simulink model "TARGET_CAN_WORKING_BUILD"  (R2023b)
settings: Solver=FixedStepAuto  StartTime=0.0  StopTime=Inf  RelTol=1e-3  EnableMultiTasking=on
InitFcn:
  | addpath('C:\MTU_DMD_CAN\COMMON_DATA'); mcb_pmsm_foc_qep_dyno_f28069m_data;
undefined symbols (not defined in the file): DiscIntNeverNeededParam, Down, GPTRIP1SEL, GPTRIP2SEL, inverter_motor1, inverter_motor2, PI_params_motor1, PI_params_motor2, pmsm_motor1, pmsm_motor2, PU_System_motor2, target, Ts, Ts_motor, Ts_speed, TZ1, TZ2, Up
libraries: simulink x11, c2802xlib x10, c280xlib x9, mcbcontrolslib x6, mcbpositiondecoderlib x6, c2806xlib x5, svdschedulerlib x3, mcbpmsmnonlinearlib x2, autolibpmsmexterior x2, mcbplantlib x2, demo_controls x1, slpidlib x1
(part 1 of 3)
settings Model: SimulationMode=external  ExtModeTrigDuration=8  Creator=The MathWorks, Inc.  LastModifiedBy=vmbasvi
settings OptimizationCC: DefaultParameterBehavior=Inlined  DefaultUnderspecifiedDataType=single  EnhancedBackFolding=on  PassReuseOutputArgsAs=Individual arguments  LifeSpan=Inf  MaxStackSize=1024  OptimizeBlockOrder=speed  DifferentSizesBufferReuse=on  OptimizationCustomize=off  EfficientTunableParamExpr=on
settings DebuggingCC: MultiTaskDSMMsg=none  ParameterPrecisionLossMsg=none  ParameterTunabilityLossMsg=error  ModelReferenceExtraNoncontSigs=none
settings HardwareCC: ProdBitPerChar=16  ProdBitPerInt=16  ProdBitPerPointer=32  ProdBitPerSizeT=32  ProdBitPerPtrDiffT=32  ProdLargestAtomicInteger=Integer  ProdLargestAtomicFloat=None  ProdWordSize=16  ProdLongLongMode=on  ProdHWDeviceType=Texas Instruments->C2000  HardwareBoardFeatureSet=SoCBlockset
settings ModelReferenceCC: ModelReferenceNumInstancesAllowed=Single
settings SFSimCC: MATLABDynamicMemAlloc=off
settings RTWCC: Description=Embedded Coder  SystemTargetFile=ert.tlc  HardwareBoard=TI Piccolo F28069M LaunchPad  TemplateMakefile=ert_default_tmf  Toolchain=Texas Instruments Code Composer Studio (C2000)  CodeProfilingSaveOptions=MetricsOnly
settings CodeAppCC: ForceParamTrailComments=on  IgnoreCustomStorageClasses=off  OperatorAnnotations=on  SimulinkDataObjDesc=on  SFDataObjDesc=on  InsertBlockDesc=on
settings ERTTargetCC: CodeReplacementLibrary=TI C28x  ParMdlRefBuildCompliant=off  CompOptLevelCompliant=off  ConcurrentExecutionCompliant=off  ExtModeTransport=4  ExtModeStaticAlloc=on  ExtModeAutomaticAllocSize=off  ExtModeStaticAllocSize=2000  ExtModeMexFile=ext_xcp  ExtModeIntrfLevel=Level2 - Open  MemSecPackage=tic2000demospkg

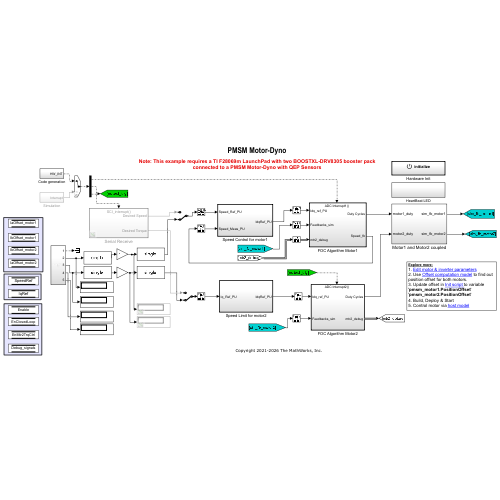
[thumbnail: Simulink's stored preview of the top-level diagram]
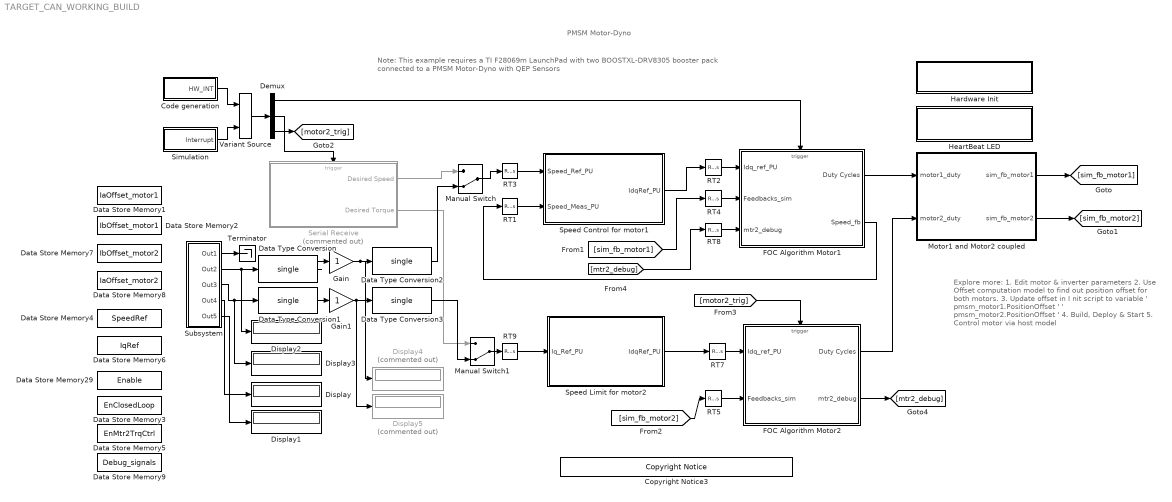
== system TARGET_CAN_WORKING_BUILD ==
  note: Explore more:
      | 1. Edit motor & inverter parameters
      | 2. Use Offset computation model to find out position offset for both motors.
      | 3. Update offset in I nit script to variable ' pmsm_motor1.PositionOffset '
      | ' pmsm_motor2.PositionOffset '
      | 4. Build, Deploy & Start
      | 5. Control motor via host model
  note: PMSM Motor-Dyno
  note: Note: This example requires a TI F28069m LaunchPad with two BOOSTXL-DRV8305 booster pack
      | connected to a PMSM Motor-Dyno with QEP Sensors
  Code generation : Subsystem
  Copyright Notice3 : demo_controls/Copyright Notice  year=2021  prod=tic2000
  Data Store Memory1 : DataStoreMemory  DataStoreName=IaOffset_motor1  ReadBeforeWriteMsg=warning  WriteAfterWriteMsg=warning  WriteAfterReadMsg=warning  InitialValue=inverter_motor1.CtSensAOffset  ShowAdditionalParam=off
  Data Store Memory2 : DataStoreMemory  DataStoreName=IbOffset_motor1  ReadBeforeWriteMsg=warning  WriteAfterWriteMsg=warning  WriteAfterReadMsg=warning  InitialValue=inverter_motor1.CtSensBOffset  ShowAdditionalParam=off
  Data Store Memory29 : DataStoreMemory  DataStoreName=Enable  ReadBeforeWriteMsg=warning  WriteAfterWriteMsg=warning  WriteAfterReadMsg=warning  ShowAdditionalParam=off  OutDataTypeStr=boolean
  Data Store Memory3 : DataStoreMemory  DataStoreName=EnClosedLoop  ReadBeforeWriteMsg=warning  WriteAfterWriteMsg=warning  WriteAfterReadMsg=warning  ShowAdditionalParam=off  OutDataTypeStr=boolean
  Data Store Memory4 : DataStoreMemory  DataStoreName=SpeedRef  ShowAdditionalParam=off
  Data Store Memory5 : DataStoreMemory  DataStoreName=EnMtr2TrqCtrl  ReadBeforeWriteMsg=warning  WriteAfterWriteMsg=warning  WriteAfterReadMsg=warning  ShowAdditionalParam=off  OutDataTypeStr=boolean
  Data Store Memory6 : DataStoreMemory  DataStoreName=IqRef  ShowAdditionalParam=off
  Data Store Memory7 : DataStoreMemory  DataStoreName=IbOffset_motor2  ReadBeforeWriteMsg=warning  WriteAfterWriteMsg=warning  WriteAfterReadMsg=warning  InitialValue=inverter_motor2.CtSensBOffset  ShowAdditionalParam=off
  Data Store Memory8 : DataStoreMemory  DataStoreName=IaOffset_motor2  ReadBeforeWriteMsg=warning  WriteAfterWriteMsg=warning  WriteAfterReadMsg=warning  InitialValue=inverter_motor2.CtSensBOffset  ShowAdditionalParam=off
  Data Store Memory9 : DataStoreMemory  DataStoreName=Debug_signals  ReadBeforeWriteMsg=warning  WriteAfterWriteMsg=warning  WriteAfterReadMsg=warning  InitialValue=5  ShowAdditionalParam=off  OutDataTypeStr=uint16
  Data Type Conversion{,1..3} (4 alike) : DataTypeConversion  OutDataTypeStr=single  SaturateOnIntegerOverflow=off  RndMeth=Floor
  Demux : Demux  Outputs=3
  Display{,1..3} (4 alike) : Display
  Display4 : Display  Commented=on
  Display5 : Display  Commented=on
  FOC Algorithm Motor1 : Subsystem
      settings: RTWSystemCode=Nonreusable function
  FOC Algorithm Motor2 : Subsystem
      settings: RTWSystemCode=Nonreusable function
  Gain : Gain
  Gain1 : Gain
  Hardware Init : Subsystem  TreatAsAtomicUnit=on
  HeartBeat LED : Subsystem
  Manual Switch : ManualSwitch  CurrentSetting=0
  Manual Switch1 : ManualSwitch  CurrentSetting=0
  Motor1 and Motor2 coupled : Subsystem
  RT1 : RateTransition  Deterministic=off  OutPortSampleTime=Ts_speed
  RT{2,4..5,7..8} (5 alike) : RateTransition  Deterministic=off
  RT3 : RateTransition  Deterministic=off  OutPortSampleTime=Ts_speed
  RT9 : RateTransition  Deterministic=off  OutPortSampleTime=Ts_speed
  Serial Receive : Subsystem  Commented=on  SystemSampleTime=1e-3
  Simulation : Subsystem
  Speed Control for motor1 : Subsystem  TreatAsAtomicUnit=on  SystemSampleTime=Ts_speed
  Speed Limit for motor2 : Subsystem  TreatAsAtomicUnit=on  SystemSampleTime=Ts_speed
  Subsystem : Subsystem
  Terminator : Terminator
  Variant Source : VariantSource  VariantControlMode=sim codegen switching  OutputFunctionCall=on
  wires:
  RT9/1 -> Speed Limit for motor2/1(Iq_Ref_PU)
  Motor1 and Motor2 coupled/2(sim_fb_motor2) -> [sim_fb_motor2]
  RT4/1 -> FOC Algorithm Motor1/2(Feedbacks_sim)
  RT7/1 -> FOC Algorithm Motor2/1(Idq_ref_PU)
  Speed Limit for motor2/1(IdqRef_PU) -> RT7/1
  Speed Control for motor1/1(IdqRef_PU) -> RT2/1
  Demux/3 -> [motor2_trig]
  [sim_fb_motor1] -> RT4/1
  RT1/1 -> Speed Control for motor1/2(Speed_Meas_PU)
  Demux/1 -> FOC Algorithm Motor1/Trigger
  [motor2_trig] -> FOC Algorithm Motor2/Trigger
  FOC Algorithm Motor2/1(Duty Cycles) -> Motor1 and Motor2 coupled/2(motor2_duty)
  Motor1 and Motor2 coupled/1(sim_fb_motor1) -> [sim_fb_motor1]
  [sim_fb_motor2] -> RT5/1
  RT5/1 -> FOC Algorithm Motor2/2(Feedbacks_sim)
  RT3/1 -> Speed Control for motor1/1(Speed_Ref_PU)
  Simulation/1(Interrupt) -> Variant Source/2
  FOC Algorithm Motor1/2(Speed_fb) -> RT1/1
  FOC Algorithm Motor1/1(Duty Cycles) -> Motor1 and Motor2 coupled/1(motor1_duty)
  Variant Source/1 -> Demux/1
  RT2/1 -> FOC Algorithm Motor1/1(Idq_ref_PU)
  Code generation/1(HW_INT) -> Variant Source/1
  Demux/2 -> Serial Receive/Trigger
  FOC Algorithm Motor2/2(mtr2_debug) -> [mtr2_debug]
  [mtr2_debug] -> RT8/1
  RT8/1 -> FOC Algorithm Motor1/3(mtr2_debug)
  Manual Switch1/1 -> RT9/1
  Subsystem/3(Out3) -> Display3/1, Data Type Conversion1/1
  Serial Receive/1(Desired Speed) -> Manual Switch/1
  Manual Switch/1 -> RT3/1
  Subsystem/2(Out2) -> Display2/1, Data Type Conversion/1
  Serial Receive/2(Desired Torque) -> Manual Switch1/1
  Subsystem/4(Out4) -> Display/1
  Subsystem/5(Out5) -> Display1/1
  Subsystem/1(Out1) -> Terminator/1
  Data Type Conversion/1 -> Gain/1
  Data Type Conversion1/1 -> Gain1/1
  Gain/1 -> Display4/1, Data Type Conversion2/1
  Data Type Conversion2/1 -> Manual Switch/2
  Gain1/1 -> Display5/1, Data Type Conversion3/1
  Data Type Conversion3/1 -> Manual Switch1/2

== system TARGET_CAN_WORKING_BUILD/Code generation ==
  HWI_ADCINT1 : svdschedulerlib/Hardware Interrupt v2  ISRGroup=ADC - Analog to Digital Converter  ISRName=ADCA1_INT  ISRNumber=32  NumEventsToServe=1  EventsList=[{'on','EOC event','1'};{'off','Overflow event','2'};{'off','Custom event','3'};{'off','Default event','4'}]  SelectedEvents={'event1'}  TaskPriority=30  DisablePreemption=off  ClearInterruptFlagsAtEndOfEvent=on  InterruptDefinitionFile=$(TARGET_ROOT)/registry/interrupts/F2837xS_interrupts.xml  HardwareBoard=F2837x  EnableSimPort=off
      settings: LibrarySourceBlock=c2000lib/Scheduling/Hardware Interrupt
  HWI_ADCINT2 : svdschedulerlib/Hardware Interrupt v2  ISRGroup=ADC - Analog to Digital Converter  ISRName=ADCA1_INT  ISRNumber=32  NumEventsToServe=1  EventsList={'on','EOC event','1';'off','Overflow event','2';'off','Custom event','3'}  SelectedEvents={'event1'}  TaskPriority=35  DisablePreemption=off  ClearInterruptFlagsAtEndOfEvent=on  InterruptDefinitionFile=$(TARGET_ROOT)/registry/interrupts/F2837xS_interrupts.xml  HardwareBoard=F2837x  EnableSimPort=off
      settings: LibrarySourceBlock=c2000lib/Scheduling/Hardware Interrupt
  HWI_SCIRXINTA : svdschedulerlib/Hardware Interrupt v2  Commented=on  ISRGroup=ADC - Analog to Digital Converter  ISRName=ADCA1_INT  ISRNumber=32  NumEventsToServe=1  EventsList={'on','EOC event','1';'off','Overflow event','2';'off','Custom event','3'}  SelectedEvents={'event1'}  TaskPriority=50  DisablePreemption=on  ClearInterruptFlagsAtEndOfEvent=on  InterruptDefinitionFile=$(TARGET_ROOT)/registry/interrupts/F2837xS_interrupts.xml  HardwareBoard=F2837x  EnableSimPort=off
      settings: LibrarySourceBlock=c2000lib/Scheduling/Hardware Interrupt
  Mux : Mux  Inputs=3
  HW_INT : Outport
  wires:
  HWI_ADCINT1/1 -> Mux/1
  HWI_SCIRXINTA/1 -> Mux/2
  HWI_ADCINT2/1 -> Mux/3
  Mux/1 -> HW_INT/1

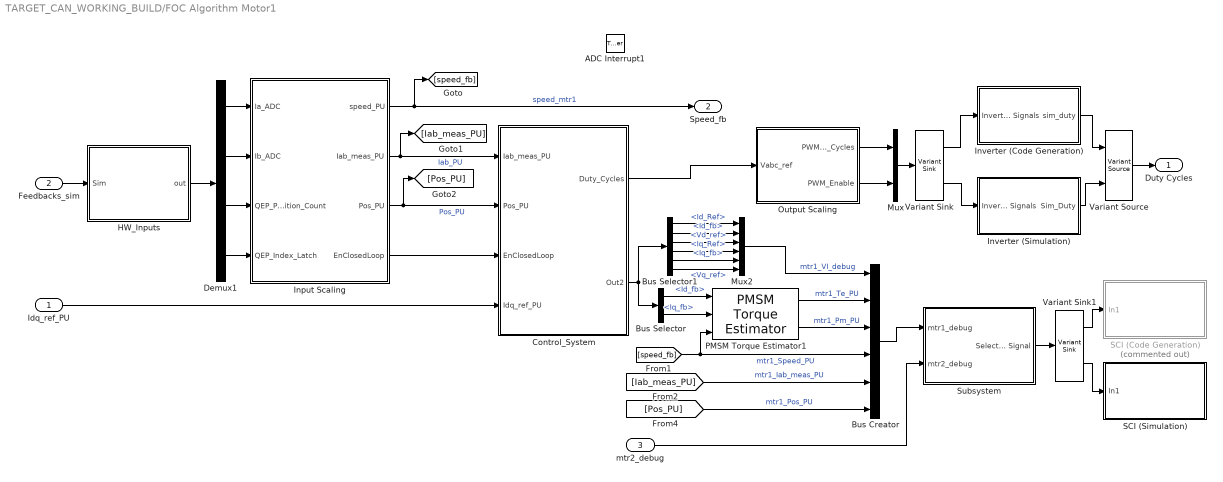
== system TARGET_CAN_WORKING_BUILD/FOC Algorithm Motor1 ==
  Idq_ref_PU : Inport
  Feedbacks_sim : Inport  Port=2
  mtr2_debug : Inport  Port=3
  ADC Interrupt1 : TriggerPort  TriggerType=function-call  VariantControl=Variant  PortDimensions=1
  Bus Creator : BusCreator  Inputs=6
  Bus Selector : BusSelector  OutputSignals=Id_fb,Iq_fb
  Bus Selector1 : BusSelector  OutputSignals=Id_Ref,Id_fb,Vd_ref,Iq_Ref,Iq_fb,Vq_ref
  Control_System : Subsystem
  Demux1 : Demux
  HW_Inputs : Subsystem  Variant=on  VariantControlMode=sim codegen switching
  Input Scaling : Subsystem
  Inverter (Code Generation) : Subsystem  VariantControl=Choice
  Inverter (Simulation) : Subsystem
  Mux : Mux  Inputs=2
  Mux2 : Mux  Inputs=6
  Output Scaling : Subsystem
  PMSM Torque Estimator1 : mcbpmsmnonlinearlib/PMSM Torque Estimator  polePairs=pmsm_motor1.p  nonLinearityChoice=Linear model with lumped parameters  Ld=pmsm_motor1.Ld  Lq=pmsm_motor1.Lq  FluxPM=pmsm_motor1.FluxPM  idVec=[-40, -20, 0, 20]  iqVec=[-40, -20, 0, 20, 40]  LdTable=0.2e-3 * ones(4, 5)  LqTable=0.2e-3 * ones(4, 5)  FluxPMTable=6.4e-3 * ones(4, 5)  FluxDTable=[-1.6,-1.6,-1.6,-1.6,-1.6;2.4,2.4,2.4,2.4,2.4;6.4,6.4,6.4,6.4,6.4;10.4,10.4,10.4,10.4,10.4]*1e-3  FluxQTable=[-8,-4,0,4,8;-8,-4,0,4,8;-8,-4,0,4,8;-8,-4,0,4,8]*1e-3  Units=Per-Unit (PU)  V_base=PU_System_motor1.V_base  I_base=PU_System_motor1.I_base  N_base=PU_System_motor1.N_base  T_base=0.90449  P_base=489.9229  scaledTables=on
  SCI (Code Generation) : Subsystem  Commented=on
  SCI (Simulation) : Subsystem
  Subsystem : Subsystem
  Variant Sink : VariantSink  VariantControlMode=sim codegen switching
  Variant Sink1 : VariantSink  VariantControlMode=sim codegen switching
  Variant Source : VariantSource  VariantControlMode=sim codegen switching
  Duty Cycles : Outport  InitialOutput=0  VectorParamsAs1DForOutWhenUnconnected=off
  Speed_fb : Outport  Port=2  InitialOutput=0  VectorParamsAs1DForOutWhenUnconnected=off
  wires:
  Control_System/1(Duty_Cycles) -> Output Scaling/1(Vabc_ref)
  Input Scaling/3(Pos_PU) -> [Pos_PU], Control_System/2(Pos_PU)  "Pos_PU"
  Idq_ref_PU/1 -> Control_System/4(Idq_ref_PU)
  Output Scaling/1(PWM_Duty_Cycles) -> Mux/1
  Variant Sink1/1 -> SCI (Code Generation)/1(In1)
  Subsystem/1(Selected Signal) -> Variant Sink1/1
  Inverter (Simulation)/1(Sim_Duty) -> Variant Source/2
  Inverter (Code Generation)/1(sim_duty) -> Variant Source/1
  Variant Sink1/2 -> SCI (Simulation)/1(In1)
  Mux/1 -> Variant Sink/1
  Variant Sink/1 -> Inverter (Code Generation)/1(Inverter Signals)
  Output Scaling/2(PWM_Enable) -> Mux/2
  Variant Source/1 -> Duty Cycles/1
  Feedbacks_sim/1 -> HW_Inputs/1(Sim)
  Input Scaling/4(EnClosedLoop) -> Control_System/3(EnClosedLoop)
  Variant Sink/2 -> Inverter (Simulation)/1(Inverter Signals)
  Input Scaling/2(Iab_meas_PU) -> [Iab_meas_PU], Control_System/1(Iab_meas_PU)  "Iab_PU"
  HW_Inputs/1(out) -> Demux1/1
  Demux1/1 -> Input Scaling/1(Ia_ADC)
  Demux1/2 -> Input Scaling/2(Ib_ADC)
  Input Scaling/1(speed_PU) -> [speed_fb], Speed_fb/1  "speed_mtr1"
  Demux1/3 -> Input Scaling/3(QEP_Position_Count)
  Demux1/4 -> Input Scaling/4(QEP_Index_Latch)
  Bus Selector1/4 -> Mux2/4  "<Iq_Ref>"
  [Iab_meas_PU] -> Bus Creator/5  "mtr1_Iab_meas_PU"
  mtr2_debug/1 -> Subsystem/2(mtr2_debug)
  Mux2/1 -> Bus Creator/1  "mtr1_VI_debug"
  Bus Selector1/6 -> Mux2/6  "<Vq_ref>"
  Bus Selector1/2 -> Mux2/2  "<Id_fb>"
  Bus Selector1/3 -> Mux2/3  "<Vd_ref>"
  Bus Selector1/1 -> Mux2/1  "<Id_Ref>"
  Bus Selector1/5 -> Mux2/5  "<Iq_fb>"
  Bus Selector/2 -> PMSM Torque Estimator1/2  "<Iq_fb>"
  Bus Creator/1 -> Subsystem/1(mtr1_debug)
  PMSM Torque Estimator1/2 -> Bus Creator/3  "mtr1_Pm_PU"
  Bus Selector/1 -> PMSM Torque Estimator1/1  "<Id_fb>"
  [speed_fb] -> PMSM Torque Estimator1/3, Bus Creator/4  "mtr1_Speed_PU"
  PMSM Torque Estimator1/1 -> Bus Creator/2  "mtr1_Te_PU"
  [Pos_PU] -> Bus Creator/6  "mtr1_Pos_PU"
  Control_System/2(Out2) -> Bus Selector/1, Bus Selector1/1

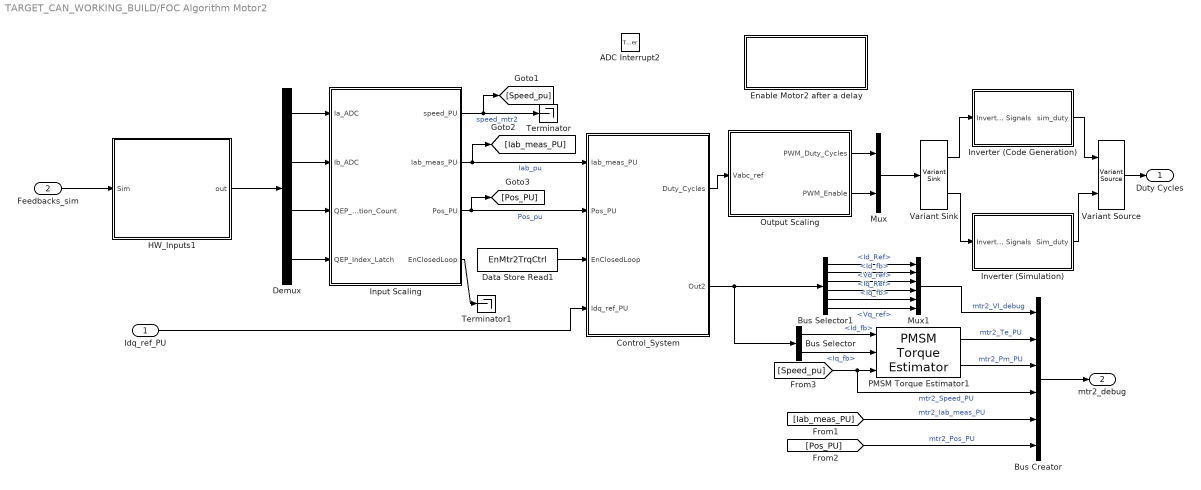
== system TARGET_CAN_WORKING_BUILD/FOC Algorithm Motor2 ==
  Idq_ref_PU : Inport
  Feedbacks_sim : Inport  Port=2
  ADC Interrupt2 : TriggerPort  TriggerType=function-call  VariantControl=Variant  PortDimensions=1
  Bus Creator : BusCreator  Inputs=6
  Bus Selector : BusSelector  OutputSignals=Id_fb,Iq_fb
  Bus Selector1 : BusSelector  OutputSignals=Id_Ref,Id_fb,Vd_ref,Iq_Ref,Iq_fb,Vq_ref
  Control_System : Subsystem
  Data Store Read1 : DataStoreRead  DataStoreName=EnMtr2TrqCtrl  IndexOptions=Index vector (dialog)  Indices=1  OutputSizes=1
  Demux : Demux
  Enable Motor2 after a delay : Subsystem  Priority=10  Variant=on  VariantControlMode=sim codegen switching
  HW_Inputs1 : Subsystem  Variant=on  VariantControlMode=sim codegen switching
  Input Scaling : Subsystem
  Inverter (Code Generation) : Subsystem  VariantControl=Choice
  Inverter (Simulation) : Subsystem
  Mux : Mux  Inputs=2
  Mux1 : Mux  Inputs=6
  Output Scaling : Subsystem
  PMSM Torque Estimator1 : mcbpmsmnonlinearlib/PMSM Torque Estimator  polePairs=pmsm_motor2.p  nonLinearityChoice=Linear model with lumped parameters  Ld=pmsm_motor2.Ld  Lq=pmsm_motor2.Lq  FluxPM=pmsm_motor2.FluxPM  idVec=[-40, -20, 0, 20]  iqVec=[-40, -20, 0, 20, 40]  LdTable=0.2e-3 * ones(4, 5)  LqTable=0.2e-3 * ones(4, 5)  FluxPMTable=6.4e-3 * ones(4, 5)  FluxDTable=[-1.6,-1.6,-1.6,-1.6,-1.6;2.4,2.4,2.4,2.4,2.4;6.4,6.4,6.4,6.4,6.4;10.4,10.4,10.4,10.4,10.4]*1e-3  FluxQTable=[-8,-4,0,4,8;-8,-4,0,4,8;-8,-4,0,4,8;-8,-4,0,4,8]*1e-3  Units=Per-Unit (PU)  V_base=PU_System_motor2.V_base  I_base=PU_System_motor2.I_base  N_base=PU_System_motor2.N_base  T_base=0.90449  P_base=489.9229  scaledTables=on
  Terminator : Terminator
  Terminator1 : Terminator
  Variant Sink : VariantSink  VariantControlMode=sim codegen switching
  Variant Source : VariantSource  VariantControlMode=sim codegen switching
  Duty Cycles : Outport  InitialOutput=0  VectorParamsAs1DForOutWhenUnconnected=off
  mtr2_debug : Outport  Port=2  VectorParamsAs1DForOutWhenUnconnected=off
  wires:
  Variant Sink/2 -> Inverter (Simulation)/1(Inverter Signals)
  Variant Source/1 -> Duty Cycles/1
  Output Scaling/2(PWM_Enable) -> Mux/2
  Variant Sink/1 -> Inverter (Code Generation)/1(Inverter Signals)
  Mux/1 -> Variant Sink/1
  Inverter (Code Generation)/1(sim_duty) -> Variant Source/1
  Inverter (Simulation)/1(Sim_duty) -> Variant Source/2
  Output Scaling/1(PWM_Duty_Cycles) -> Mux/1
  Input Scaling/2(Iab_meas_PU) -> Control_System/1(Iab_meas_PU), [Iab_meas_PU]  "Iab_pu"
  Input Scaling/3(Pos_PU) -> Control_System/2(Pos_PU), [Pos_PU]  "Pos_pu"
  Control_System/1(Duty_Cycles) -> Output Scaling/1(Vabc_ref)
  Data Store Read1/1 -> Control_System/3(EnClosedLoop)
  Feedbacks_sim/1 -> HW_Inputs1/1(Sim)
  Input Scaling/4(EnClosedLoop) -> Terminator1/1
  Input Scaling/1(speed_PU) -> [Speed_pu], Terminator/1  "speed_mtr2"
  Demux/1 -> Input Scaling/1(Ia_ADC)
  Demux/2 -> Input Scaling/2(Ib_ADC)
  HW_Inputs1/1(out) -> Demux/1
  Idq_ref_PU/1 -> Control_System/4(Idq_ref_PU)
  Demux/3 -> Input Scaling/3(QEP_Position_Count)
  Demux/4 -> Input Scaling/4(QEP_Index_Latch)
  Bus Selector1/5 -> Mux1/5  "<Iq_fb>"
  [Speed_pu] -> Bus Creator/4, PMSM Torque Estimator1/3  "mtr2_Speed_PU"
  [Iab_meas_PU] -> Bus Creator/5  "mtr2_Iab_meas_PU"
  Bus Selector1/4 -> Mux1/4  "<Iq_Ref>"
  Mux1/1 -> Bus Creator/1  "mtr2_VI_debug"
  Bus Selector1/2 -> Mux1/2  "<Id_fb>"
  [Pos_PU] -> Bus Creator/6  "mtr2_Pos_PU"
  Bus Selector1/1 -> Mux1/1  "<Id_Ref>"
  Bus Selector1/6 -> Mux1/6  "<Vq_ref>"
  Bus Selector/2 -> PMSM Torque Estimator1/2  "<Iq_fb>"
  Bus Creator/1 -> mtr2_debug/1
  PMSM Torque Estimator1/2 -> Bus Creator/3  "mtr2_Pm_PU"
  PMSM Torque Estimator1/1 -> Bus Creator/2  "mtr2_Te_PU"
  Bus Selector/1 -> PMSM Torque Estimator1/1  "<Id_fb>"
  Bus Selector1/3 -> Mux1/3  "<Vd_ref>"
  Control_System/2(Out2) -> Bus Selector/1, Bus Selector1/1

== system TARGET_CAN_WORKING_BUILD/Hardware Init ==
  Event Listener : EventListener  DisableCoverage=on  EventName=reset
  HW_Init : Subsystem  Variant=on  VariantControlMode=sim codegen switching

== system TARGET_CAN_WORKING_BUILD/HeartBeat LED ==
  Constant : Constant  OutDataTypeStr=uint16  SampleTime=0.5
  LED blink : c2806xlib/Digital Output  GPIO_Number=GPIO32~GPIO39  GPIO_Bit0=off  GPIO_BIT0_Toggle=off  GPIO_Bit1=off  GPIO_BIT1_Toggle=off  GPIO_Bit2=on  GPIO_BIT2_Toggle=on  GPIO_Bit3=off  GPIO_BIT3_Toggle=off  GPIO_Bit4=off  GPIO_BIT4_Toggle=off  GPIO_Bit5=off  GPIO_BIT5_Toggle=off  GPIO_Bit6=off  GPIO_BIT6_Toggle=off  GPIO_Bit7=off  GPIO_BIT7_Toggle=on
  wires:
  Constant/1 -> LED blink/1

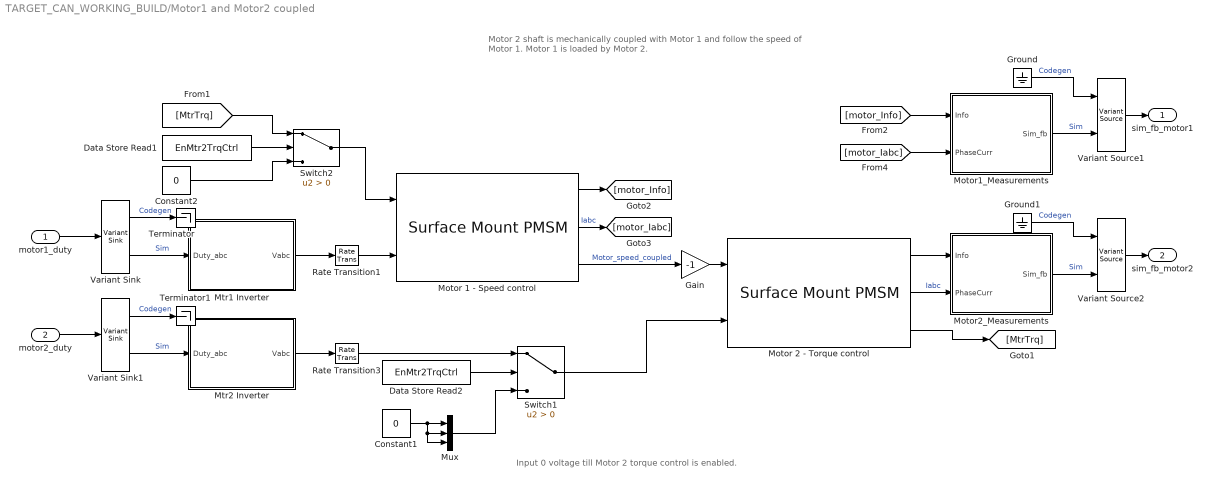
== system TARGET_CAN_WORKING_BUILD/Motor1 and Motor2 coupled ==
  note: Motor 2 shaft is mechanically coupled with Motor 1
      | and follow the speed of Motor 1.
      |
      | Motor 1 is loaded by Motor 2.
  note: Input 0 voltage till Motor 2 torque control is enabled.
  motor1_duty : Inport
  motor2_duty : Inport  Port=2
  Constant1 : Constant  Value=0
  Constant2 : Constant  Value=0
  Data Store Read1 : DataStoreRead  DataStoreName=EnMtr2TrqCtrl  IndexOptions=Index vector (dialog)  Indices=1  OutputSizes=1
  Data Store Read2 : DataStoreRead  DataStoreName=EnMtr2TrqCtrl  IndexOptions=Index vector (dialog)  Indices=1  OutputSizes=1
  Gain : Gain  Gain=-1
  Ground : Ground
  Ground1 : Ground
  Motor 1 - Speed control : autolibpmsmexterior/Surface Mount PMSM  port_config=Torque  sim_type=Discrete  Ts=Ts_motor  P=pmsm_motor1.p  Rs=pmsm_motor1.Rs  Ldq_=pmsm_motor1.Ld  KConstText=Permanent flux linkage constant (lambda_pm):  lambda_pm=pmsm_motor1.FluxPM  Ke=159.9771  Kt=1.323  mechanical=[pmsm_motor1.J, pmsm_motor1.B, 0]  idq0=[0 0]  theta_init=0  omega_init=0  KConst=pmsm_motor1.FluxPM  lambda_pm_calc=pmsm_motor1.FluxPM  RefBlkName='autolibpmsmexterior/Surface Mount PMSM'  aMode=5  Ldq="[0.0002      0.0002]"
  Motor 2 - Torque control : autolibpmsmexterior/Surface Mount PMSM  port_config=Speed  sim_type=Discrete  Ts=Ts_motor  P=pmsm_motor2.p  Rs=pmsm_motor2.Rs  Ldq_=pmsm_motor2.Ld  KConstText=Permanent flux linkage constant (lambda_pm):  lambda_pm=pmsm_motor2.FluxPM  Ke=159.9771  Kt=1.323  mechanical=[0.0027, 4.924e-4, 0]  idq0=[0 0]  theta_init=0  omega_init=0  KConst=pmsm_motor2.FluxPM  lambda_pm_calc=pmsm_motor2.FluxPM  RefBlkName='autolibpmsmexterior/Surface Mount PMSM'  aMode=5  Ldq="[0.0002      0.0002]"
  Motor1_Measurements : Subsystem
  Motor2_Measurements : Subsystem
  Mtr1 Inverter : Subsystem
  Mtr2 Inverter : Subsystem
  Mux : Mux  Inputs=3
  Rate Transition1 : RateTransition  Deterministic=off  OutPortSampleTime=Ts_motor
  Rate Transition3 : RateTransition  Integrity=off  OutPortSampleTime=Ts_motor
  Switch1 : Switch  Criteria=u2 > Threshold  SaturateOnIntegerOverflow=off  InputSameDT=off
  Switch2 : Switch  Criteria=u2 > Threshold  SaturateOnIntegerOverflow=off  InputSameDT=off
  Terminator : Terminator
  Terminator1 : Terminator
  Variant Sink : VariantSink  VariantControlMode=sim codegen switching
  Variant Sink1 : VariantSink  VariantControlMode=sim codegen switching
  Variant Source1 : VariantSource  VariantControlMode=sim codegen switching
  Variant Source2 : VariantSource  VariantControlMode=sim codegen switching
  sim_fb_motor1 : Outport  VectorParamsAs1DForOutWhenUnconnected=off
  sim_fb_motor2 : Outport  Port=2  VectorParamsAs1DForOutWhenUnconnected=off
  wires:
  motor1_duty/1 -> Variant Sink/1
  Variant Source1/1 -> sim_fb_motor1/1
  Motor1_Measurements/1(Sim_fb) -> Variant Source1/2  "Sim"
  Ground/1 -> Variant Source1/1  "Codegen"
  Variant Sink/1 -> Terminator/1  "Codegen"
  Rate Transition1/1 -> Motor 1 - Speed control/2
  Mtr1 Inverter/1(Vabc) -> Rate Transition1/1
  Motor 1 - Speed control/3 -> Gain/1  "Motor_speed_coupled"
  [motor_Info] -> Motor1_Measurements/1(Info)
  [motor_Iabc] -> Motor1_Measurements/2(PhaseCurr)
  Motor 1 - Speed control/1 -> [motor_Info]
  Motor 1 - Speed control/2 -> [motor_Iabc]  "Iabc"
  Motor 2 - Torque control/1 -> Motor2_Measurements/1(Info)
  Motor 2 - Torque control/2 -> Motor2_Measurements/2(PhaseCurr)  "Iabc"
  Motor2_Measurements/1(Sim_fb) -> Variant Source2/2  "Sim"
  Mtr2 Inverter/1(Vabc) -> Rate Transition3/1
  Motor 2 - Torque control/3 -> [MtrTrq]
  Variant Sink/2 -> Mtr1 Inverter/1(Duty_abc)  "Sim"
  Variant Sink1/2 -> Mtr2 Inverter/1(Duty_abc)  "Sim"
  Ground1/1 -> Variant Source2/1  "Codegen"
  Variant Source2/1 -> sim_fb_motor2/1
  motor2_duty/1 -> Variant Sink1/1
  Variant Sink1/1 -> Terminator1/1  "Codegen"
  Gain/1 -> Motor 2 - Torque control/1
  Switch2/1 -> Motor 1 - Speed control/1
  Rate Transition3/1 -> Switch1/1
  Constant2/1 -> Switch2/3
  Data Store Read1/1 -> Switch2/2
  [MtrTrq] -> Switch2/1
  Switch1/1 -> Motor 2 - Torque control/2
  Mux/1 -> Switch1/3
  Data Store Read2/1 -> Switch1/2
  Constant1/1 -> Mux/2, Mux/3, Mux/1

== system TARGET_CAN_WORKING_BUILD/Serial Receive ==
  SCI_interrupt : TriggerPort  TriggerType=function-call  VariantControl=Variant  PortDimensions=1
  Code Generation : Subsystem
  Data Store Write : DataStoreWrite  DataStoreName=Enable  IndexOptions=Index vector (dialog)  Indices=1  OutputSizes=1
  Data Store Read1 : DataStoreRead  DataStoreName=IqRef  IndexOptions=Index vector (dialog)  Indices=1  OutputSizes=1
  Data Store Read2 : DataStoreRead  DataStoreName=SpeedRef  IndexOptions=Index vector (dialog)  Indices=1  OutputSizes=1
  Data Type Conversion3 : DataTypeConversion  OutDataTypeStr=boolean  RndMeth=Simplest  SaturateOnIntegerOverflow=off
  Reference Signal : Subsystem
  Simulation : Subsystem  VariantControl=(sim)
  Variant Source : VariantSource  VariantControlMode=sim codegen switching
  Desired Speed : Outport
  Desired Torque : Outport  Port=2
  wires:
  Data Store Read1/1 -> Desired Torque/1
  Data Store Read2/1 -> Desired Speed/1
  Data Type Conversion3/1 -> Data Store Write/1
  Code Generation/1(Data) -> Reference Signal/1(In1)
  Reference Signal/1(Enable_PWM) -> Variant Source/1
  Simulation/1(Enable_PWM) -> Variant Source/2
  Variant Source/1 -> Data Type Conversion3/1

== system TARGET_CAN_WORKING_BUILD/Simulation ==
  Mux : Mux  Inputs=3
  Pulse Generator1 : DiscretePulseGenerator  PulseType=Time based  Period=Ts  PulseWidth=20  PhaseDelay=Ts
  Pulse Generator2 : DiscretePulseGenerator  PulseType=Time based  Period=Ts  PulseWidth=20
  SCI_Rx_INT : simulink/Ports & Subsystems/Function-Call Generator  sample_time=0.1  numberOfIterations=1  DisallowWideOutput=off
  Simulation1 : Subsystem
  Simulation2 : Subsystem
  Interrupt : Outport
  wires:
  Pulse Generator1/1 -> Simulation1/Trigger
  Mux/1 -> Interrupt/1
  Simulation1/1(Interrupt) -> Mux/3
  SCI_Rx_INT/1 -> Mux/2
  Pulse Generator2/1 -> Simulation2/Trigger
  Simulation2/1(Interrupt) -> Mux/1

== system TARGET_CAN_WORKING_BUILD/Speed Control for motor1 ==
  Speed_Ref_PU : Inport
  Speed_Meas_PU : Inport  Port=2
  Id_ref : Constant  Value=0  OutDataTypeStr=dataType  SampleTime=Ts_speed
  Mux1 : Mux  Inputs=2
  PI_Controller_Speed : Subsystem
  Speed_Ref_Selector : Subsystem
  IdqRef_PU : Outport  VectorParamsAs1DForOutWhenUnconnected=off
  wires:
  Speed_Meas_PU/1 -> Speed_Ref_Selector/2(Speed_Ref_Open), PI_Controller_Speed/2(N_fb)  "Speed_fb"
  Id_ref/1 -> Mux1/1
  PI_Controller_Speed/1(Iq_ref) -> Mux1/2
  Mux1/1 -> IdqRef_PU/1
  Speed_Ref_Selector/1(Speed_Ref_PU) -> PI_Controller_Speed/1(N_ref)  "Speed_Ref"
  Speed_Ref_PU/1 -> Speed_Ref_Selector/1(Speed_Ref_In)

== system TARGET_CAN_WORKING_BUILD/Speed Limit for motor2 ==
  Iq_Ref_PU : Inport
  IIR Filter : mcbcontrolslib/IIR Filter  VariantControl=Low Pass Filter  VariantSelect=Low-pass  Filter_constant=0.01  advancedSettings=off  Ts=50e-6  cutOff_freq=32.1525
  Id_ref_PU : Constant  Value=0  OutDataTypeStr=dataType
  Mux1 : Mux  Inputs=2
  IdqRef_PU : Outport  VectorParamsAs1DForOutWhenUnconnected=off
  wires:
  Iq_Ref_PU/1 -> Mux1/2
  Id_ref_PU/1 -> Mux1/1
  Mux1/1 -> IIR Filter/1
  IIR Filter/1 -> IdqRef_PU/1

== system TARGET_CAN_WORKING_BUILD/Subsystem ==
  Byte Unpack : svdutilitieslib/Byte Unpack  dimensions={[1],[1],[1],[1]}  datatypes={'uint16','uint16','uint16','uint16'}  byteAlign=2  blockPlatform=tic2000
      settings: LibrarySourceBlock=c2000lib/Target Communication/Byte Unpack
  CAN Receive : c280xlib/CAN Receive  chipFamily=C280x  useModule=CAN_A  mailboxNo=0  messageID=256  messageType=Standard (11-bit identifier)  enableAcceptanceFiltering=off  messageIDMask=0  sampleTime=0.03  dataType=uint16  outputAction=Output last received values  initValue=0  outputMessageID=off  outputMessageLength=off  outputMessageTimeStamp=off  postInterrupt=off  interruptLine=0
      settings: LibrarySourceBlock=c2806xlib/CAN Receive
  Data Type Conversion : DataTypeConversion  OutDataTypeStr=single  SaturateOnIntegerOverflow=off  RndMeth=Floor
  Data Type Conversion1 : DataTypeConversion  OutDataTypeStr=single  SaturateOnIntegerOverflow=off  RndMeth=Floor
  Display : Display
  Display1 : Display
  Out1 : Outport
  Out2 : Outport  Port=2
  Out3 : Outport  Port=3
  Out4 : Outport  Port=4
  Out5 : Outport  Port=5
  wires:
  Byte Unpack/4 -> Out5/1, Display1/1
  Byte Unpack/1 -> Data Type Conversion/1
  Data Type Conversion1/1 -> Out3/1
  Byte Unpack/2 -> Data Type Conversion1/1
  CAN Receive/1 -> Out1/1
  CAN Receive/2 -> Byte Unpack/1
  Byte Unpack/3 -> Out4/1, Display/1
  Data Type Conversion/1 -> Out2/1

== system TARGET_CAN_WORKING_BUILD/FOC Algorithm Motor1/Control_System ==
  Iab_meas_PU : Inport
  Pos_PU : Inport  Port=2
  EnClosedLoop : Inport  Port=3
  Idq_ref_PU : Inport  Port=4
  Closed loop Control : Subsystem
  Data Store Read : DataStoreRead  DataStoreName=Enable  IndexOptions=Index vector (dialog)  Indices=1  OutputSizes=1
  Data Store Write : DataStoreWrite  DataStoreName=EnClosedLoop  IndexOptions=Index vector (dialog)  Indices=1  OutputSizes=1
  NOT : Logic  Operator=NOT  IconShape=distinctive  AllPortsSameDT=off  OutDataTypeStr=boolean
  Open Loop Start-Up : Subsystem
  Switch : Switch  Criteria=u2 > Threshold  Threshold=0.5  SaturateOnIntegerOverflow=off  InputSameDT=off
  Duty_Cycles : Outport  VectorParamsAs1DForOutWhenUnconnected=off
  Out2 : Outport  Port=2
  wires:
  Iab_meas_PU/1 -> Closed loop Control/1(Iab_meas_PU)
  Pos_PU/1 -> Closed loop Control/2(Pos_PU)
  Idq_ref_PU/1 -> Closed loop Control/3(Idq_ref_PU)
  Closed loop Control/1(Vabc in PU) -> Switch/1
  Switch/1 -> Duty_Cycles/1
  EnClosedLoop/1 -> Closed loop Control/Enable, Data Store Write/1, NOT/1, Switch/2
  Open Loop Start-Up/1(PWM_Duty) -> Switch/3
  NOT/1 -> Open Loop Start-Up/Enable
  Data Store Read/1 -> Closed loop Control/4(EnablePWM)
  Closed loop Control/2(Idq_debug) -> Out2/1

== system TARGET_CAN_WORKING_BUILD/FOC Algorithm Motor1/HW_Inputs ==
  Sim : Inport
  Sensor Driver Blocks (codegen) : Subsystem  VariantControl=(codegen)
  Sensor Driver Blocks (sim) : Subsystem  VariantControl=(sim)
  out : Outport

== system TARGET_CAN_WORKING_BUILD/FOC Algorithm Motor1/Input Scaling ==
  note: Current Measurements
  Ia_ADC : Inport
  Ib_ADC : Inport  Port=2
  QEP_Position_Count : Inport  Port=3
  QEP_Index_Latch : Inport  Port=4
  " Calculate Speed" : Subsystem
  Calculate Phase Currents : Subsystem
  Constant : Constant  Value=pmsm_motor1.PositionOffset  OutDataTypeStr=dataType  SampleTime=-1
  speed_PU : Outport
  Iab_meas_PU : Outport  Port=2
  Pos_PU : Outport  Port=3
  EnClosedLoop : Outport  Port=4
  wires:
  " Calculate Speed"/2(speed) -> speed_PU/1
  Calculate Phase Currents/1(Iab_meas_PU) -> Iab_meas_PU/1  "Iab_fb_PU"
  QEP_Position_Count/1 -> " Calculate Speed"/1(QEP_Position_Count)
  " Calculate Speed"/1(Theta_e) -> Pos_PU/1
  Ia_ADC/1 -> Calculate Phase Currents/1(Ia_ADC)
  Ib_ADC/1 -> Calculate Phase Currents/2(Ib_ADC)
  Constant/1 -> " Calculate Speed"/3(Offset)
  QEP_Index_Latch/1 -> " Calculate Speed"/2(QEP_Index_Latch)
  " Calculate Speed"/3(IndexFound) -> EnClosedLoop/1

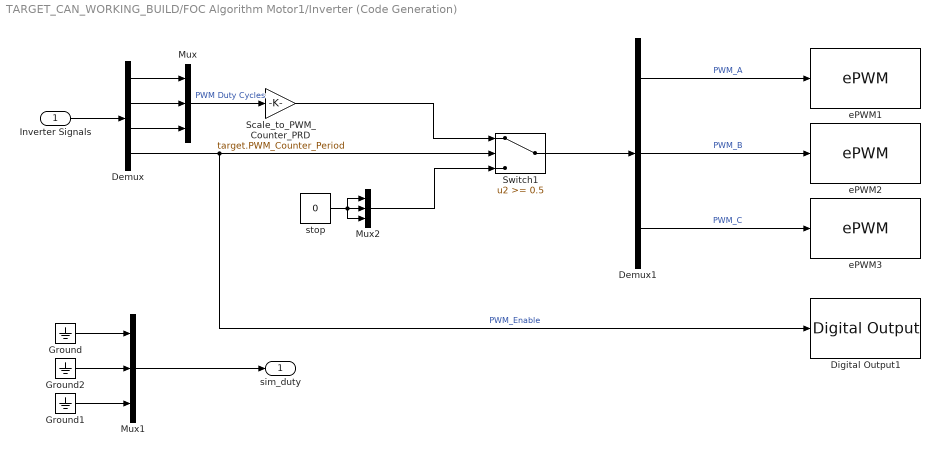
== system TARGET_CAN_WORKING_BUILD/FOC Algorithm Motor1/Inverter (Code Generation) ==
  Inverter Signals : Inport
  Demux : Demux
  Demux1 : Demux  Outputs=3
  Digital Output1 : c2806xlib/Digital Output  GPIO_Number=GPIO50~GPIO55  GPIO_Bit0=off  GPIO_BIT0_Toggle=off  GPIO_Bit1=off  GPIO_BIT1_Toggle=off  GPIO_Bit2=on  GPIO_BIT2_Toggle=off  GPIO_Bit3=off  GPIO_BIT3_Toggle=off  GPIO_Bit4=off  GPIO_BIT4_Toggle=off  GPIO_Bit5=off  GPIO_BIT5_Toggle=off  GPIO_Bit6=off  GPIO_BIT6_Toggle=off  GPIO_Bit7=off  GPIO_BIT7_Toggle=off
  Ground : Ground
  Ground1 : Ground
  Ground2 : Ground
  Mux : Mux  Inputs=3
  Mux1 : Mux  Inputs=3
  Mux2 : Mux  Inputs=3
  Scale_to_PWM_Counter_PRD : Gain  Gain=target.PWM_Counter_Period  OutDataTypeStr=uint16  RndMeth=Simplest
  Switch1 : Switch  Threshold=0.5  SaturateOnIntegerOverflow=off  InputSameDT=off
  ePWM1 : c2802xlib/ePWM  PwmType=C2000  useModule=ePWM1  ePWMxLINKTBPRD=Not Linked  periodUnits=Clock cycles  timerSource=Specify via dialog  timerPeriod_clk=target.PWM_Counter_Period+1  timerPeriod_sec=64000  tbshadow=Counter equals to zero  countingMode=Up-Down  phaseActiveEnable=Disable  phaseDirection=Count down after sync  phaseActive=0  synchronizationEnable=off  dcaevt1Sync=off  dcbevt1Sync=off  synchronizationOption=Counter equals to zero (CTR=Zero)  dcbevt1SyncOut=off  dcaevt1SyncOut=off  cmpdSyncOut=off  cmpcSyncOut=off  cmpbSyncOut=off  zeroSyncOut=on  swfSyncOut=off  perSynchronizationOption=Counter equals to period (CTR=PRD)  clockPrescale=1  HSclockPrescale=1  enswap=off  ePWMxAStatus=on  ePWMxAactionLogic1=Do nothing  ePWMxAactionLogic2=Do nothing  ePWMxAactionLogic3=Clear  ePWMxAactionLogic4=Set  ePWMxAactionLogic5=Do nothing  ePWMxAactionLogic6=Do nothing  ePWMxACSFenable=off  ePWMxACSFvalue=Forcing disable  ePWMxASFreload=Zero  ePWMxBStatus=off  ePWMxBactionLogic1=Do nothing  ePWMxBactionLogic2=Set  ePWMxBactionLogic3=Do nothing  ePWMxBactionLogic4=Do nothing  ePWMxBactionLogic5=Clear  ePWMxBactionLogic6=Do nothing  ePWMxBCSFenable=off  ePWMxBCSFvalue=Forcing disable  ePWMxBSFreload=Zero  ePWNxBOutWay=off  ePWMxLINKCMPA=Not Linked  CMPAUnits=Clock cycles  CMPASource=Input port  CMPAValue_per=32000  CMPAValue_clk=target.PWM_Counter_Period/2+1  enCMPAshadow=Counter equals to zero (CTR=Zero)  ePWMxLINKCMPB=Not Linked  CMPBUnits=Clock cycles  CMPBSource=Specify via dialog  CMPBValue_per=50  CMPBValue_clk=target.PWM_Counter_Period/2+1  enCMPBshadow=Counter equals to zero (CTR=Zero)  ePWMxLINKCMPC=Not Linked  CMPCUnits=Clock cycles  CMPCSource=Specify via dialog  CMPCValue_per=50  CMPCValue_clk=32000  enCMPCshadow=Counter equals to zero (CTR=Zero)  ePWMxLINKCMPD=Not Linked  CMPDUnits=Clock cycles  CMPDSource=Specify via dialog  CMPDValue_per=50  CMPDValue_clk=32000  enCMPDshadow=Counter equals to zero (CTR=Zero)  enableDBePWMxA=on  enableDBePWMxB=on  enhalfcycle=off  DBpolarity=Active high complementary (AHC)  DBedgeDelay=Positive  DBSource_ePWMxA=ePWMxA  DBSource_ePWMxB=ePWMxA  DBPeriodUnits=Clock cycles  DBperiodSource=Specify via dialog  REDperiod=15  FEDperiod=15  REDperiod_sec=0  FEDperiod_sec=0  LoadModeDBRED=Immediate without using shadow  LoadModeDBFED=Immediate without using shadow  adcstartModuleA=on  adcrequestEventA=First event  adcstartEventA=Counter equals to period (CTR=PRD)  adcstartEventA_type2=Digital Compare Module A Event 1 start of conversion (DCAEVT1.soc)  adcstartModuleB=off  adcrequestEventB=First event  adcstartEventB=Counter equals to zero (CTR=Zero)  adcstartEventB_type2=Counter equals to zero (CTR=Zero)  intEn=off  intPrd=First event  intSel=Counter equals to zero (CTR=Zero)  intSel_type2=Counter equals to zero (CTR=Zero)  hrpe=off  enHRPWM=off  HRPWM_LoadMode=Counter equals to period (CTR=PRD)  HRPWM_CTLMode=Duty or Period control mode  HRPWM_EDGMode=Both edge  hrpeb=off  enHRPWMB=off  HRPWM_LoadModeB=Counter equals to zero (CTR=ZERO)  HRPWM_CTLModeB=Duty or Period control mode  HRPWM_EDGModeB=Both edge  enHRDBRED=off  enHRDBFED=off  enSFO=on  enautoconv=on  chopperEnable=off  chopperFrequency=1  chopperFirstwidth=1  chopperDuty=12.5%  tripZonesource=Specify via dialog  tzselOSHT1=off  tzselOSHT2=off  tzselOSHT3=off  tzselOSHDCAEV1=off  tzselOSHDCBEV1=off  tzselCBC1=off  tzselCBC2=off  tzselCBC3=off  tzselCBCDCAEV2=off  tzselCBCDCBEV2=off  tzselOSHT4=off  tzselOSHT5=off  tzselOSHT6=off  tzselCBC4=off  tzselCBC5=off  tzselCBC6=off  enTzOstIntr=off  enTzCbcIntr=off  enTzDCAEVT1Intr=off  enTzDCAEVT2Intr=off  enTzDCBEVT1Intr=off  enTzDCBEVT2Intr=off  ePWMxAforced=No action  ePWMxBforced=No action  DCAEVT1forced=No action  DCBEVT1forced=No action  DCAEVT2forced=No action  DCBEVT2forced=No action  dcah=Trip Zone 1 input (TZ1)  dcal=Trip Zone 2 input (TZ2)  dcbh=Trip Zone 1 input (TZ1)  dcbl=Trip Zone 2 input (TZ2)  dcah_type2=GPTRIP1SEL/(TZ1)  dcal_type2=GPTRIP2SEL/(TZ2)  dcbh_type2=GPTRIP1SEL/(TZ1)  dcbl_type2=GPTRIP2SEL/(TZ2)  gendcaevt1=Event disabled  gendcaevt2=Event disabled  gendcbevt1=Event disabled  gendcbevt2=Event disabled  dcaevt1src=DCAEVT1 with sync  dcaevt2src=DCAEVT2 with sync  dcbevt1src=DCBEVT1 with sync  dcbevt2src=DCBEVT2 with sync  pulsesel=Counter equals to zero (CTR=Zero)  blankinv=off  blankoffset=0  blankwidth=0  evsrcsel=Filtered version of DCAEVT1 (DCAEVT1FILT)  encape=off
  ePWM2 : c2802xlib/ePWM  PwmType=C2000  useModule=ePWM2  ePWMxLINKTBPRD=Not Linked  periodUnits=Clock cycles  timerSource=Specify via dialog  timerPeriod_clk=target.PWM_Counter_Period+1  timerPeriod_sec=64000  tbshadow=Counter equals to zero  countingMode=Up-Down  phaseActiveEnable=Set counter to phase value specified via dialog  phaseDirection=Count up after sync  phaseActive=0  synchronizationEnable=off  dcaevt1Sync=off  dcbevt1Sync=off  synchronizationOption=Pass through (EPWMxSYNCI or SWFSYNC)  dcbevt1SyncOut=off  dcaevt1SyncOut=off  cmpdSyncOut=off  cmpcSyncOut=off  cmpbSyncOut=off  zeroSyncOut=off  swfSyncOut=on  perSynchronizationOption=Counter equals to period (CTR=PRD)  clockPrescale=1  HSclockPrescale=1  enswap=off  ePWMxAStatus=on  ePWMxAactionLogic1=Do nothing  ePWMxAactionLogic2=Do nothing  ePWMxAactionLogic3=Clear  ePWMxAactionLogic4=Set  ePWMxAactionLogic5=Do nothing  ePWMxAactionLogic6=Do nothing  ePWMxACSFenable=off  ePWMxACSFvalue=Forcing disable  ePWMxASFreload=Zero  ePWMxBStatus=off  ePWMxBactionLogic1=Do nothing  ePWMxBactionLogic2=Set  ePWMxBactionLogic3=Do nothing  ePWMxBactionLogic4=Do nothing  ePWMxBactionLogic5=Clear  ePWMxBactionLogic6=Do nothing  ePWMxBCSFenable=off  ePWMxBCSFvalue=Forcing disable  ePWMxBSFreload=Zero  ePWNxBOutWay=off  ePWMxLINKCMPA=Not Linked  CMPAUnits=Clock cycles  CMPASource=Input port  CMPAValue_per=32000  CMPAValue_clk=target.PWM_Counter_Period/2+1  enCMPAshadow=Counter equals to zero (CTR=Zero)  ePWMxLINKCMPB=Not Linked  CMPBUnits=Clock cycles  CMPBSource=Specify via dialog  CMPBValue_per=50  CMPBValue_clk=target.PWM_Counter_Period/2+1  enCMPBshadow=Counter equals to zero (CTR=Zero)  ePWMxLINKCMPC=Not Linked  CMPCUnits=Clock cycles  CMPCSource=Specify via dialog  CMPCValue_per=50  CMPCValue_clk=32000  enCMPCshadow=Counter equals to zero (CTR=Zero)  ePWMxLINKCMPD=Not Linked  CMPDUnits=Clock cycles  CMPDSource=Specify via dialog  CMPDValue_per=50  CMPDValue_clk=32000  enCMPDshadow=Counter equals to zero (CTR=Zero)  enableDBePWMxA=on  enableDBePWMxB=on  enhalfcycle=off  DBpolarity=Active high complementary (AHC)  DBedgeDelay=Positive  DBSource_ePWMxA=ePWMxA  DBSource_ePWMxB=ePWMxA  DBPeriodUnits=Clock cycles  DBperiodSource=Specify via dialog  REDperiod=15  FEDperiod=15  REDperiod_sec=0  FEDperiod_sec=0  LoadModeDBRED=Immediate without using shadow  LoadModeDBFED=Immediate without using shadow  adcstartModuleA=off  adcrequestEventA=First event  adcstartEventA=Digital Compare Module A Event 1 start of conversion (DCAEVT1.soc)  adcstartEventA_type2=Digital Compare Module A Event 1 start of conversion (DCAEVT1.soc)  adcstartModuleB=off  adcrequestEventB=First event  adcstartEventB=Counter equals to zero (CTR=Zero)  adcstartEventB_type2=Counter equals to zero (CTR=Zero)  intEn=off  intPrd=First event  intSel=Counter equals to zero (CTR=Zero)  intSel_type2=Counter equals to zero (CTR=Zero)  hrpe=off  enHRPWM=off  HRPWM_LoadMode=Counter equals to period (CTR=PRD)  HRPWM_CTLMode=Duty or Period control mode  HRPWM_EDGMode=Both edge  hrpeb=off  enHRPWMB=off  HRPWM_LoadModeB=Counter equals to zero (CTR=ZERO)  HRPWM_CTLModeB=Duty or Period control mode  HRPWM_EDGModeB=Both edge  enHRDBRED=off  enHRDBFED=off  enSFO=on  enautoconv=on  chopperEnable=off  chopperFrequency=1  chopperFirstwidth=1  chopperDuty=12.5%  tripZonesource=Specify via dialog  tzselOSHT1=off  tzselOSHT2=off  tzselOSHT3=off  tzselOSHDCAEV1=off  tzselOSHDCBEV1=off  tzselCBC1=off  tzselCBC2=off  tzselCBC3=off  tzselCBCDCAEV2=off  tzselCBCDCBEV2=off  tzselOSHT4=off  tzselOSHT5=off  tzselOSHT6=off  tzselCBC4=off  tzselCBC5=off  tzselCBC6=off  enTzOstIntr=off  enTzCbcIntr=off  enTzDCAEVT1Intr=off  enTzDCAEVT2Intr=off  enTzDCBEVT1Intr=off  enTzDCBEVT2Intr=off  ePWMxAforced=No action  ePWMxBforced=No action  DCAEVT1forced=No action  DCBEVT1forced=No action  DCAEVT2forced=No action  DCBEVT2forced=No action  dcah=Trip Zone 1 input (TZ1)  dcal=Trip Zone 2 input (TZ2)  dcbh=Trip Zone 1 input (TZ1)  dcbl=Trip Zone 2 input (TZ2)  dcah_type2=GPTRIP1SEL/(TZ1)  dcal_type2=GPTRIP2SEL/(TZ2)  dcbh_type2=GPTRIP1SEL/(TZ1)  dcbl_type2=GPTRIP2SEL/(TZ2)  gendcaevt1=Event disabled  gendcaevt2=Event disabled  gendcbevt1=Event disabled  gendcbevt2=Event disabled  dcaevt1src=DCAEVT1 with sync  dcaevt2src=DCAEVT2 with sync  dcbevt1src=DCBEVT1 with sync  dcbevt2src=DCBEVT2 with sync  pulsesel=Counter equals to zero (CTR=Zero)  blankinv=off  blankoffset=0  blankwidth=0  evsrcsel=Filtered version of DCAEVT1 (DCAEVT1FILT)  encape=off
  ePWM3 : c2802xlib/ePWM  PwmType=C2000  useModule=ePWM3  ePWMxLINKTBPRD=Not Linked  periodUnits=Clock cycles  timerSource=Specify via dialog  timerPeriod_clk=target.PWM_Counter_Period+1  timerPeriod_sec=64000  tbshadow=Counter equals to zero  countingMode=Up-Down  phaseActiveEnable=Set counter to phase value specified via dialog  phaseDirection=Count up after sync  phaseActive=0  synchronizationEnable=off  dcaevt1Sync=off  dcbevt1Sync=off  synchronizationOption=Pass through (EPWMxSYNCI or SWFSYNC)  dcbevt1SyncOut=off  dcaevt1SyncOut=off  cmpdSyncOut=off  cmpcSyncOut=off  cmpbSyncOut=off  zeroSyncOut=off  swfSyncOut=on  perSynchronizationOption=Counter equals to period (CTR=PRD)  clockPrescale=1  HSclockPrescale=1  enswap=off  ePWMxAStatus=on  ePWMxAactionLogic1=Do nothing  ePWMxAactionLogic2=Do nothing  ePWMxAactionLogic3=Clear  ePWMxAactionLogic4=Set  ePWMxAactionLogic5=Do nothing  ePWMxAactionLogic6=Do nothing  ePWMxACSFenable=off  ePWMxACSFvalue=Forcing disable  ePWMxASFreload=Zero  ePWMxBStatus=off  ePWMxBactionLogic1=Do nothing  ePWMxBactionLogic2=Set  ePWMxBactionLogic3=Do nothing  ePWMxBactionLogic4=Do nothing  ePWMxBactionLogic5=Clear  ePWMxBactionLogic6=Do nothing  ePWMxBCSFenable=off  ePWMxBCSFvalue=Forcing disable  ePWMxBSFreload=Zero  ePWNxBOutWay=off  ePWMxLINKCMPA=Not Linked  CMPAUnits=Clock cycles  CMPASource=Input port  CMPAValue_per=32000  CMPAValue_clk=target.PWM_Counter_Period/2+1  enCMPAshadow=Counter equals to zero (CTR=Zero)  ePWMxLINKCMPB=Not Linked  CMPBUnits=Clock cycles  CMPBSource=Specify via dialog  CMPBValue_per=50  CMPBValue_clk=target.PWM_Counter_Period/2+1  enCMPBshadow=Counter equals to zero (CTR=Zero)  ePWMxLINKCMPC=Not Linked  CMPCUnits=Clock cycles  CMPCSource=Specify via dialog  CMPCValue_per=50  CMPCValue_clk=32000  enCMPCshadow=Counter equals to zero (CTR=Zero)  ePWMxLINKCMPD=Not Linked  CMPDUnits=Clock cycles  CMPDSource=Specify via dialog  CMPDValue_per=50  CMPDValue_clk=32000  enCMPDshadow=Counter equals to zero (CTR=Zero)  enableDBePWMxA=on  enableDBePWMxB=on  enhalfcycle=off  DBpolarity=Active high complementary (AHC)  DBedgeDelay=Positive  DBSource_ePWMxA=ePWMxA  DBSource_ePWMxB=ePWMxA  DBPeriodUnits=Clock cycles  DBperiodSource=Specify via dialog  REDperiod=15  FEDperiod=15  REDperiod_sec=0  FEDperiod_sec=0  LoadModeDBRED=Immediate without using shadow  LoadModeDBFED=Immediate without using shadow  adcstartModuleA=off  adcrequestEventA=First event  adcstartEventA=Digital Compare Module A Event 1 start of conversion (DCAEVT1.soc)  adcstartEventA_type2=Digital Compare Module A Event 1 start of conversion (DCAEVT1.soc)  adcstartModuleB=off  adcrequestEventB=First event  adcstartEventB=Counter equals to zero (CTR=Zero)  adcstartEventB_type2=Counter equals to zero (CTR=Zero)  intEn=off  intPrd=First event  intSel=Counter equals to zero (CTR=Zero)  intSel_type2=Counter equals to zero (CTR=Zero)  hrpe=off  enHRPWM=off  HRPWM_LoadMode=Counter equals to period (CTR=PRD)  HRPWM_CTLMode=Duty or Period control mode  HRPWM_EDGMode=Both edge  hrpeb=off  enHRPWMB=off  HRPWM_LoadModeB=Counter equals to zero (CTR=ZERO)  HRPWM_CTLModeB=Duty or Period control mode  HRPWM_EDGModeB=Both edge  enHRDBRED=off  enHRDBFED=off  enSFO=on  enautoconv=on  chopperEnable=off  chopperFrequency=1  chopperFirstwidth=1  chopperDuty=12.5%  tripZonesource=Specify via dialog  tzselOSHT1=off  tzselOSHT2=off  tzselOSHT3=off  tzselOSHDCAEV1=off  tzselOSHDCBEV1=off  tzselCBC1=off  tzselCBC2=off  tzselCBC3=off  tzselCBCDCAEV2=off  tzselCBCDCBEV2=off  tzselOSHT4=off  tzselOSHT5=off  tzselOSHT6=off  tzselCBC4=off  tzselCBC5=off  tzselCBC6=off  enTzOstIntr=off  enTzCbcIntr=off  enTzDCAEVT1Intr=off  enTzDCAEVT2Intr=off  enTzDCBEVT1Intr=off  enTzDCBEVT2Intr=off  ePWMxAforced=No action  ePWMxBforced=No action  DCAEVT1forced=No action  DCBEVT1forced=No action  DCAEVT2forced=No action  DCBEVT2forced=No action  dcah=Trip Zone 1 input (TZ1)  dcal=Trip Zone 2 input (TZ2)  dcbh=Trip Zone 1 input (TZ1)  dcbl=Trip Zone 2 input (TZ2)  dcah_type2=GPTRIP1SEL/(TZ1)  dcal_type2=GPTRIP2SEL/(TZ2)  dcbh_type2=GPTRIP1SEL/(TZ1)  dcbl_type2=GPTRIP2SEL/(TZ2)  gendcaevt1=Event disabled  gendcaevt2=Event disabled  gendcbevt1=Event disabled  gendcbevt2=Event disabled  dcaevt1src=DCAEVT1 with sync  dcaevt2src=DCAEVT2 with sync  dcbevt1src=DCBEVT1 with sync  dcbevt2src=DCBEVT2 with sync  pulsesel=Counter equals to zero (CTR=Zero)  blankinv=off  blankoffset=0  blankwidth=0  evsrcsel=Filtered version of DCAEVT1 (DCAEVT1FILT)  encape=off
  stop : Constant  Value=0  OutDataTypeStr=uint16
  sim_duty : Outport  VectorParamsAs1DForOutWhenUnconnected=off
  wires:
  Demux1/3 -> ePWM3/1  "PWM_C"
  Scale_to_PWM_Counter_PRD/1 -> Switch1/1
  Mux2/1 -> Switch1/3
  stop/1 -> Mux2/3, Mux2/2, Mux2/1
  Demux/4 -> Switch1/2, Digital Output1/1  "PWM_Enable"
  Inverter Signals/1 -> Demux/1
  Demux1/2 -> ePWM2/1  "PWM_B"
  Switch1/1 -> Demux1/1
  Demux1/1 -> ePWM1/1  "PWM_A"
  Mux/1 -> Scale_to_PWM_Counter_PRD/1  "PWM Duty Cycles"
  Ground/1 -> Mux1/1
  Ground1/1 -> Mux1/3
  Ground2/1 -> Mux1/2
  Mux1/1 -> sim_duty/1
  Demux/1 -> Mux/1
  Demux/2 -> Mux/2
  Demux/3 -> Mux/3

== system TARGET_CAN_WORKING_BUILD/FOC Algorithm Motor1/Inverter (Simulation) ==
  Inverter Signals : Inport
  Data Type Duplicate : DataTypeDuplicate
  Demux : Demux
  Mux : Mux  Inputs=3
  Mux2 : Mux  Inputs=3
  Switch1 : Switch  Threshold=0.5  RndMeth=Simplest  SaturateOnIntegerOverflow=off  InputSameDT=off
  stop : Constant  Value=0  OutDataTypeStr=Inherit: Inherit via back propagation
  Sim_Duty : Outport  VectorParamsAs1DForOutWhenUnconnected=off
  wires:
  stop/1 -> Data Type Duplicate/2, Mux2/1, Mux2/3, Mux2/2
  Mux2/1 -> Switch1/3
  Switch1/1 -> Sim_Duty/1
  Inverter Signals/1 -> Demux/1
  Demux/4 -> Switch1/2  "PWM Enable"
  Mux/1 -> Data Type Duplicate/1, Switch1/1  "PWM Duty Cycles"
  Demux/1 -> Mux/1
  Demux/2 -> Mux/2
  Demux/3 -> Mux/3

== system TARGET_CAN_WORKING_BUILD/FOC Algorithm Motor1/Output Scaling ==
  Vabc_ref : Inport
  Constant : Constant  Value=0.5  OutDataTypeStr=dataType  SampleTime=-1
  Data Type Conversion : DataTypeConversion  OutDataTypeStr=dataType  SaturateOnIntegerOverflow=off  RndMeth=Floor
  Enable : DataStoreRead  DataStoreName=Enable  IndexOptions=Index vector (dialog)  Indices=1  OutputSizes=1
  One_by_Two : Gain  Gain=0.5  RndMeth=Simplest  OutDataTypeStr=Inherit: Same as input
  Sum : Sum  Inputs=|++
  PWM_Duty_Cycles : Outport
  PWM_Enable : Outport  Port=2
  wires:
  Constant/1 -> Sum/2
  Vabc_ref/1 -> One_by_Two/1
  Sum/1 -> PWM_Duty_Cycles/1  "Mtr1_PWM_Duty_Cycles"
  Enable/1 -> Data Type Conversion/1  "PWM_En"
  One_by_Two/1 -> Sum/1
  Data Type Conversion/1 -> PWM_Enable/1

== system TARGET_CAN_WORKING_BUILD/FOC Algorithm Motor1/SCI (Code Generation) ==
  In1 : Inport
  Data_Logging : Subsystem
  Demux : Demux  Outputs=2
  Demux2 : Demux  Outputs=2
  While Iterator Subsystem : Subsystem  TreatAsAtomicUnit=on
  wires:
  Demux2/2 -> While Iterator Subsystem/2(Iteration)  "SCI_Tx_Iteration"
  Demux2/1 -> While Iterator Subsystem/1(Data)  "SCI_Tx_Data"
  Data_Logging/1(SCI_Tx) -> Demux2/1
  Demux/1 -> Data_Logging/1(Data_Log1)
  Demux/2 -> Data_Logging/2(Data_Log2)
  In1/1 -> Demux/1

== system TARGET_CAN_WORKING_BUILD/FOC Algorithm Motor1/SCI (Simulation) ==
  In1 : Inport
  Demux : Demux  Outputs=2
  Terminator1 : Terminator
  Terminator2 : Terminator
  wires:
  In1/1 -> Demux/1
  Demux/1 -> Terminator1/1
  Demux/2 -> Terminator2/1
